simulink model "CC_M3"  (R2017b)
settings: Solver=VariableStepAuto  StartTime=0.0  StopTime=10.0  RelTol=1e-3
undefined symbols (not defined in the file): DiscIntNeverNeededParam, Kdec, KInc, Kp, Kp1

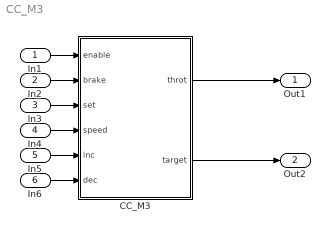
== system CC_M3 ==
  In1 : Inport
  In2 : Inport  Port=2
  In3 : Inport  Port=3
  In4 : Inport  Port=4
  In5 : Inport  Port=5
  In6 : Inport  Port=6
  CC_M3 : Subsystem
  Out1 : Outport
  Out2 : Outport  Port=2
  wires:
  CC_M3/1(throt) -> Out1/1
  In5/1 -> CC_M3/5(inc)
  In1/1 -> CC_M3/1(enable)
  In4/1 -> CC_M3/4(speed)
  CC_M3/2(target) -> Out2/1
  In3/1 -> CC_M3/3(set)
  In2/1 -> CC_M3/2(brake)
  In6/1 -> CC_M3/6(dec)

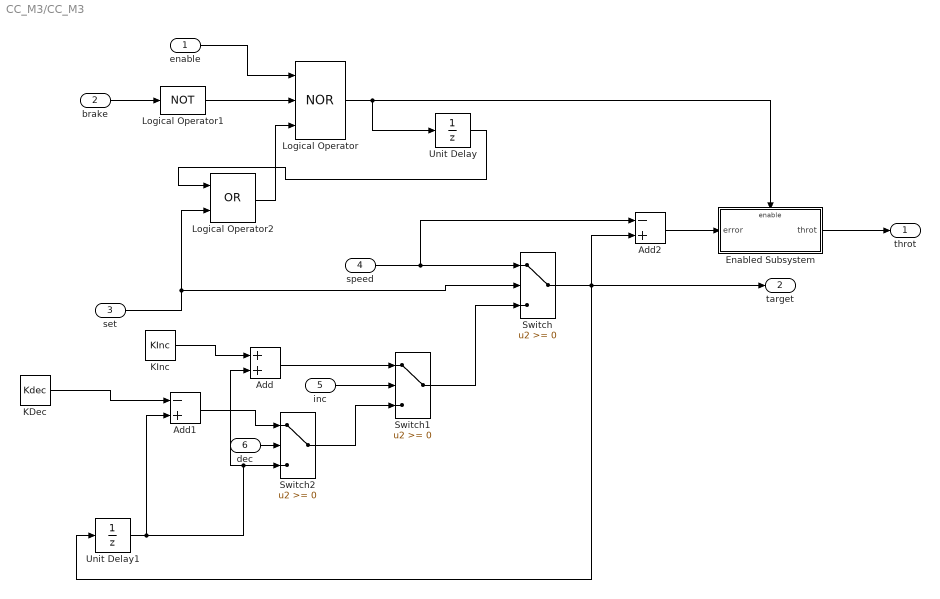
== system CC_M3/CC_M3 ==
  enable : Inport
  brake : Inport  Port=2
  set : Inport  Port=3
  speed : Inport  Port=4
  inc : Inport  Port=5
  dec : Inport  Port=6
  Add : Sum
  Add1 : Sum  Inputs=-+
  Add2 : Sum  Inputs=-+
  Enabled Subsystem : Subsystem  TreatAsAtomicUnit=on
  KDec : Constant  Value=Kdec
  KInc : Constant  Value=KInc
  Logical Operator : Logic  Operator=NOR  Inputs=3  AllPortsSameDT=off  OutDataTypeStr=boolean
  Logical Operator1 : Logic  Operator=NOT  Inputs=3  AllPortsSameDT=off  OutDataTypeStr=boolean
  Logical Operator2 : Logic  Operator=OR  AllPortsSameDT=off  OutDataTypeStr=boolean
  Switch : Switch
  Switch1 : Switch
  Switch2 : Switch
  Unit Delay : UnitDelay  InitialCondition=1  SampleTime=-1
  Unit Delay1 : UnitDelay  SampleTime=-1
  throt : Outport
  target : Outport  Port=2
  wires:
  Enabled Subsystem/1(throt) -> throt/1
  Add2/1 -> Enabled Subsystem/1(error)
  KDec/1 -> Add1/1
  Add1/1 -> Switch2/1
  KInc/1 -> Add/1
  Unit Delay1/1 -> Switch2/3, Add/2, Add1/2
  Switch/1 -> Unit Delay1/1, Add2/2, target/1
  dec/1 -> Switch2/2
  inc/1 -> Switch1/2
  Add/1 -> Switch1/1
  Switch2/1 -> Switch1/3
  Switch1/1 -> Switch/3
  speed/1 -> Switch/1, Add2/1
  Logical Operator2/1 -> Logical Operator/3
  Unit Delay/1 -> Logical Operator2/1
  Logical Operator/1 -> Unit Delay/1, Enabled Subsystem/Enable
  set/1 -> Switch/2, Logical Operator2/2
  brake/1 -> Logical Operator1/1
  Logical Operator1/1 -> Logical Operator/2
  enable/1 -> Logical Operator/1

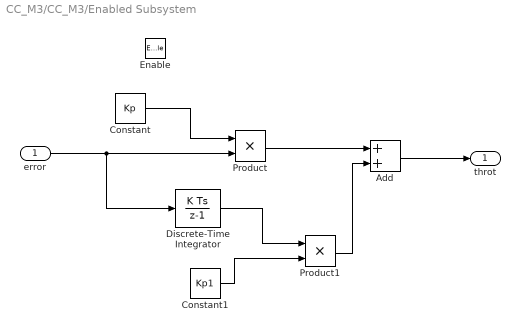
== system CC_M3/CC_M3/Enabled Subsystem ==
  error : Inport
  Enable : EnablePort
  Add : Sum
  Constant : Constant  Value=Kp
  Constant1 : Constant  Value=Kp1
  Discrete-Time Integrator : DiscreteIntegrator  gainval=Ki  ICPrevOutput=DiscIntNeverNeededParam  ICPrevScaledInput=DiscIntNeverNeededParam
  Product : Product
  Product1 : Product
  throt : Outport
  wires:
  error/1 -> Product/2, Discrete-Time Integrator/1
  Discrete-Time Integrator/1 -> Product1/1
  Product1/1 -> Add/2
  Constant1/1 -> Product1/2
  Add/1 -> throt/1
  Product/1 -> Add/1
  Constant/1 -> Product/1
